simulink model "sim_tase_2025_att_ctrl"  (R2020a)
settings: Solver=ode4  StartTime=0.0  StopTime=30.0  FixedStep=0.01  RelTol=1e-3
values from neighbouring files (symbols this model uses):
  alfa_i_init = zeros(3, NF)    [init_tase_2025_att_ctrl.m]
  beta_ij_init = zeros(3, NF)    [init_tase_2025_att_ctrl.m]
  c1 = 2.5    [init_tase_2025_att_ctrl.m]
  c1_diff_sigma_bar_w = diag([12; 12; 12])    [init_tase_2025_att_ctrl.m]
  c1_diff_ui = diag([25; 30; 20])    [init_tase_2025_att_ctrl.m]
  c2 = 2.0    (= 2)    [init_tase_2025_att_ctrl.m]
  c2_diff_sigma_bar_w = diag([12; 12; 12])    [init_tase_2025_att_ctrl.m]
  c2_diff_ui = diag([50; 50; 10])    [init_tase_2025_att_ctrl.m]
  c3_diff_sigma_bar_w = diag([15; 15; 15])    [init_tase_2025_att_ctrl.m]
  c3_diff_ui = diag([15; 15; 10])    [init_tase_2025_att_ctrl.m]
  dw_aa_t = 0.2 * ones(3, 5) + ( 1.0 - 0.2 ) * rand(3, 5)    [init_tase_2025_att_ctrl.m]
  dw_ff_t = [ 0.4 * ones(1, 5) + ( 1.0 - 0.4 ) * rand(1, 5);                      0.4 * ones(1, 5) + ( 1.0 - 0.4 ) * rand(1, 5);                      0.2 * ones(1, 5) + ( 0.6 - 0.2 ) * rand(1, 5) ]    [init_tase_2025_att_ctrl.m]
  dw_phi_t = ( - pi / 2 ) * ones(3, 5) + ( pi / 2 - ( - pi / 2 ) ) * rand(3, 5)    [init_tase_2025_att_ctrl.m]
  dwci_init = zeros(3,5)    [init_tase_2025_att_ctrl.m]
  err_wi_init = zeros(3, NF)    [init_tase_2025_att_ctrl.m]
  eta_1_ij_init = zeros(3, NF)    [init_tase_2025_att_ctrl.m]
  eta_2_ij_init = zeros(3, NF)    [init_tase_2025_att_ctrl.m]
  h1w = diag([20.0; 20.0; 20.0])    [init_tase_2025_att_ctrl.m]
  h2w = diag([30.0; 35.0; 35.0])    [init_tase_2025_att_ctrl.m]
  h3w = diag([30.0; 25.0; 30.0])    [init_tase_2025_att_ctrl.m]
  Ji = zeros(3,3,NF)    [init_tase_2025_att_ctrl.m]
  k_1_ij_hat_init = zeros(3, NF)    [init_tase_2025_att_ctrl.m]
  k_1_ij_init = zeros(3, NF)    [init_tase_2025_att_ctrl.m]
  k_1_ij_lower = zeros(3, NF)    [init_tase_2025_att_ctrl.m]
  k_1_ij_upper = zeros(3, NF)    [init_tase_2025_att_ctrl.m]
  k_2_ij_init = zeros(3, NF)    [init_tase_2025_att_ctrl.m]
  k_2_ij_lower = zeros(3, NF)    [init_tase_2025_att_ctrl.m]
  k_2_ij_upper = zeros(3, NF)    [init_tase_2025_att_ctrl.m]
  Lamd_diff_sigma_bar_w = 0.8    [init_tase_2025_att_ctrl.m]
  Lamd_diff_ui = 0.8    [init_tase_2025_att_ctrl.m]
  mu1 = 0.2    [init_tase_2025_att_ctrl.m]
  mu2 = 0.2    [init_tase_2025_att_ctrl.m]
  mu_d_w = 100    [init_tase_2025_att_ctrl.m]
  phi_ij_init = ones(3, NF)    [init_tase_2025_att_ctrl.m]
  pos0 = zeros(3, 1)    [init_tase_2025_att_ctrl.m]
  PZ0 = P0(3)    [init_tase_2025_att_ctrl.m]
  PZ1 = 10    [init_tase_2025_att_ctrl.m]
  q_ij_hat_init = zeros(3, NF)    [init_tase_2025_att_ctrl.m]
  Qci_init = repmat([1;0;0;0],1,NF)    [init_tase_2025_att_ctrl.m]
  R0 = 4    [init_tase_2025_att_ctrl.m]
  R1 = 8    [init_tase_2025_att_ctrl.m]
  Rci_init = zeros(3,3,NF)    [init_tase_2025_att_ctrl.m]
  Ri_init = zeros(3,3,NF)    [init_tase_2025_att_ctrl.m]
  Rx2 = 10    [init_tase_2025_att_ctrl.m]
  Ry2 = 6    [init_tase_2025_att_ctrl.m]
  Rz2 = 4    [init_tase_2025_att_ctrl.m]
  T0 = 0    [init_tase_2025_att_ctrl.m]
  T1 = tseq1    (= 10)    [init_tase_2025_att_ctrl.m]
  T2 = tseq1 + tseq12 + tseq2    (= 30)    [init_tase_2025_att_ctrl.m]
  T_ij = repmat([60.0; 60.0; 60.0], 1, NF)    [init_tase_2025_att_ctrl.m]
  ui_init = zeros(3,NF)    [init_tase_2025_att_ctrl.m]
  vel0 = zeros(3, 1)    [init_tase_2025_att_ctrl.m]
  wci_init = zeros(3,5)    [init_tase_2025_att_ctrl.m]
  zeta_diff_sigma_bar_w = 0.3    [init_tase_2025_att_ctrl.m]
  zeta_diff_ui = 0.05    [init_tase_2025_att_ctrl.m]
undefined symbols (not defined in the file or in its folder): cal_frac_squ, p_alfaw1, p_alfaw2, q_alfaw1, q_alfaw2, Qei_init, Qi_init, Rei_init, V_Phi_Rei_init, wei_init, wi_init
(part 3 of 5)

== matlab function sim_tase_2025_att_ctrl/cal wci dwci agent 5 ==
  data: ui_vec input; wci output; duihat_vec input; d2uihat_vec input; Rci_mat input; dwci output
function [wci, dwci] = fcn(ui_vec, duihat_vec, d2uihat_vec, Rci_mat)
%%%% 计算姿态角速率指令及其导数

iiuav = 5;
ui = ui_vec(:,iiuav);
duihat = duihat_vec(:,iiuav);
d2uihat = d2uihat_vec(:,iiuav);
Rci = Rci_mat(:,:,iiuav);

ee1 = [1;0;0];
ee2 = [0;1;0];
ee3 = [0;0;1];
RciE3 = ui / norm(ui,2);
PiMat = eye(3,3) - ee3*(ee3');
dRciE3 = (1 / norm(ui,2))*Rci*PiMat*(Rci')*duihat;
Themat = [-RciE3(2)/(1+RciE3(3)),         -RciE3(1)/(1+RciE3(3)),       (RciE3(1)*RciE3(2))/((1+RciE3(3))^2); ...
                   2*RciE3(1)/(1+RciE3(3)),                0,                               1 - (RciE3(1)^2)/((1+RciE3(3))^2); ...
                               0                                       -1                                                        0                                   ];
wcxe3 = (1 / norm(ui,2))*PiMat*(Rci')*duihat;
wcxe2 = (1 / norm(ui,2))*(Rci')*Themat*Rci*PiMat*(Rci')*duihat;
wci = [-wcxe3(2); wcxe3(1); -wcxe2(1)];

TempMat1 = [0,                           -1/(1+RciE3(3)),                   (RciE3(2))/((1+RciE3(3))^2); ...
                       2/(1+RciE3(3)),                0,                               (-2*RciE3(1))/((1+RciE3(3))^2); ...
                       0,                                     0,                                                   0                             ];
TempMat2 = [-1/(1+RciE3(3)),              0,                               (RciE3(1))/((1+RciE3(3))^2); ...
                       0,                                     0,                                                   0                      ; ...
                       0,                                     0,                                                   0                             ];
TempMat3 = [(RciE3(2))/((1+RciE3(3))^2),                 (RciE3(1))/((1+RciE3(3))^2),       (-2*RciE3(1)*RciE3(2))/((1+RciE3(3))^3); ...
                       (-2*RciE3(1))/((1+RciE3(3))^2),                             0,                               (2*(RciE3(1)^2))/((1+RciE3(3))^3); ...
                        0,                                                                          0,                                                   0                             ];
dTheMat = TempMat1*dRciE3*(ee1') + TempMat2*dRciE3*(ee2') + TempMat3*dRciE3*(ee3');
wcix = cal_askew_mat(wci);
dRciT = -wcix*(Rci');
dwcxe3 = (1 / norm(ui,2))*PiMat*(dRciT*duihat+(Rci')*(d2uihat-(((ui')*duihat)/(norm(ui,2)^2))*duihat));
dwcxe2 = (1 / norm(ui,2))*((dRciT*Themat+(Rci')*dTheMat) ...
                *(Rci*PiMat*(Rci'))*duihat + (Rci')*Themat*(Rci*PiMat*(Rci'))*(d2uihat-(((ui')*duihat)/(norm(ui,2)^2))*duihat));
dwci = [-dwcxe3(2);  dwcxe3(1);  -dwcxe2(1)];

== matlab function sim_tase_2025_att_ctrl/cal alfa_i agent 1 ==
  data: c1 input; alfa_i_1 output; Qi_vec input; eta_1_ij_vec input
function alfa_i_1 = fcn(c1, Qi_vec, eta_1_ij_vec)
%%%% 计算虚拟控制量
iiuav = 1;
alfa_i_1 = -c1 * inv( (1/2) * ( Qi_vec(1,iiuav) * eye(3) + cal_askew_mat( Qi_vec(2:4,iiuav) ) ) ) * eta_1_ij_vec(:,iiuav);

== matlab function sim_tase_2025_att_ctrl/cal alfa_i agent 2 ==
  data: c1 input; alfa_i_2 output; Qi_vec input; eta_1_ij_vec input
function alfa_i_2 = fcn(c1, Qi_vec, eta_1_ij_vec)
%%%% 计算虚拟控制量
iiuav = 2;
alfa_i_2 = -c1 * inv( (1/2) * ( Qi_vec(1,iiuav) * eye(3) + cal_askew_mat( Qi_vec(2:4,iiuav) ) ) ) * eta_1_ij_vec(:,iiuav);

== matlab function sim_tase_2025_att_ctrl/cal alfa_i agent 3 ==
  data: c1 input; alfa_i_3 output; Qi_vec input; eta_1_ij_vec input
function alfa_i_3 = fcn(c1, Qi_vec, eta_1_ij_vec)
%%%% 计算虚拟控制量
iiuav = 3;
alfa_i_3 = -c1 * inv( (1/2) * ( Qi_vec(1,iiuav) * eye(3) + cal_askew_mat( Qi_vec(2:4,iiuav) ) ) ) * eta_1_ij_vec(:,iiuav);

== matlab function sim_tase_2025_att_ctrl/cal alfa_i agent 4 ==
  data: c1 input; alfa_i_4 output; Qi_vec input; eta_1_ij_vec input
function alfa_i_4 = fcn(c1, Qi_vec, eta_1_ij_vec)
%%%% 计算虚拟控制量
iiuav = 4;
alfa_i_4 = -c1 * inv( (1/2) * ( Qi_vec(1,iiuav) * eye(3) + cal_askew_mat( Qi_vec(2:4,iiuav) ) ) ) * eta_1_ij_vec(:,iiuav);

== matlab function sim_tase_2025_att_ctrl/cal alfa_i agent 5 ==
  data: c1 input; alfa_i_5 output; Qi_vec input; eta_1_ij_vec input
function alfa_i_5 = fcn(c1, Qi_vec, eta_1_ij_vec)
%%%% 计算虚拟控制量
iiuav = 5;
alfa_i_5 = -c1 * inv( (1/2) * ( Qi_vec(1,iiuav) * eye(3) + cal_askew_mat( Qi_vec(2:4,iiuav) ) ) ) * eta_1_ij_vec(:,iiuav);

== matlab function sim_tase_2025_att_ctrl/combine alfa_i ==
  data: alfa_i_1 input; alfa_i_vec output; alfa_i_2 input; alfa_i_3 input; alfa_i_4 input; alfa_i_5 input
function alfa_i_vec = fcn(alfa_i_1, alfa_i_2, alfa_i_3, alfa_i_4, alfa_i_5)
%%%% 合并预设性能函数
alfa_i_vec = [alfa_i_1(:), alfa_i_2(:), alfa_i_3(:), alfa_i_4(:), alfa_i_5(:)];

== matlab function sim_tase_2025_att_ctrl/cal phi_ij agent 1 ==
  data: tsim input; phi_ij_1 output; T_ij input
function phi_ij_1 = fcn(tsim, T_ij)
%%%% 计算性能调节函数
iiuav = 1;
phi_ij_1 = zeros(3,1);
for jj = 1:3

%     kk_phi = 1.0;
%     phi_ij_1(jj) = 1 - sin( (pi/2) * ( ( kk_phi * tsim ) / ( T_ij(jj, iiuav) ) ) );
%     if phi_ij_1(jj) < 0
%         phi_ij_1(jj) = 0;
%     end


    kk_phi = 1.0;
    if tsim <= T_ij(jj, iiuav)
        phi_ij_1(jj) = 1 - sin( (pi/2) * ( ( kk_phi * tsim ) / ( T_ij(jj, iiuav) ) ) );
    else
        phi_ij_1(jj) = 0;
    end

end

== matlab function sim_tase_2025_att_ctrl/combine wci dwci ==
  data: wci_node_1 input; wci_vec output; wci_node_2 input; wci_node_3 input; wci_node_4 input; wci_node_5 input; dwci_vec output; dwci_node_1 input; dwci_node_2 input; dwci_node_3 input; dwci_node_4 input; dwci_node_5 input
function [wci_vec, dwci_vec] = fcn(wci_node_1, wci_node_2, wci_node_3, wci_node_4, wci_node_5, ...
                                                                dwci_node_1, dwci_node_2, dwci_node_3, dwci_node_4, dwci_node_5)
%%%% 合并姿态角速率指令及其导数
wci_vec = [wci_node_1(:), wci_node_2(:), wci_node_3(:), wci_node_4(:), wci_node_5(:)];
dwci_vec = [dwci_node_1(:), dwci_node_2(:), dwci_node_3(:), dwci_node_4(:), dwci_node_5(:)];

== matlab function sim_tase_2025_att_ctrl/cal abs 11 ==
  data: x input; y output
function y = fcn(x)
y = abs(x(:));

== matlab function sim_tase_2025_att_ctrl/cal abs 12 ==
  data: x input; y output
function y = fcn(x)
y = abs(x(:));

== matlab function sim_tase_2025_att_ctrl/cal abs 13 ==
  data: x input; y output
function y = fcn(x)
y = abs(x(:));

== matlab function sim_tase_2025_att_ctrl/cal abs 14 ==
  data: x input; y output
function y = fcn(x)
y = abs(x(:));

== matlab function sim_tase_2025_att_ctrl/cal abs 15 ==
  data: x input; y output
function y = fcn(x)
y = abs(x(:));

== matlab function sim_tase_2025_att_ctrl/cal abs 16 ==
  data: x input; y output
function y = fcn(x)
y = abs(x(:));

== matlab function sim_tase_2025_att_ctrl/cal abs 17 ==
  data: x input; y output
function y = fcn(x)
y = abs(x(:));

== matlab function sim_tase_2025_att_ctrl/cal abs 18 ==
  data: x input; y output
function y = fcn(x)
y = abs(x(:));

== matlab function sim_tase_2025_att_ctrl/combine tau ==
  data: tau_1 input; taui_vec output; tau_2 input; tau_3 input; tau_4 input; tau_5 input
function taui_vec = fcn(tau_1, tau_2, tau_3, tau_4, tau_5)
%%%% 合并辅助姿态角速率
taui_vec = [tau_1(:), tau_2(:), tau_3(:), tau_4(:), tau_5(:)];

== matlab function sim_tase_2025_att_ctrl/cal phi_ij agent 2 ==
  data: tsim input; phi_ij_2 output; T_ij input
function phi_ij_2 = fcn(tsim, T_ij)
%%%% 计算性能调节函数
iiuav = 2;
phi_ij_2 = zeros(3,1);
for jj = 1:3
%     kk_phi = 1.0;
%     phi_ij_2(jj) = 1 - sin( (pi/2) * ( ( kk_phi * tsim ) / ( T_ij(jj, iiuav) ) ) );
%     if phi_ij_2(jj) < 0
%         phi_ij_2(jj) = 0;
%     end

    kk_phi = 1.0;
    if tsim <= T_ij(jj, iiuav)
        phi_ij_2(jj) = 1 - sin( (pi/2) * ( ( kk_phi * tsim ) / ( T_ij(jj, iiuav) ) ) );
    else
        phi_ij_2(jj) = 0;
    end

end

== matlab function sim_tase_2025_att_ctrl/wi dynam agent 1 ==
  data: Ji input; dwi_1 output; wi_vec input; taui_vec input; dw_vec input
function dwi_1 = fcn(Ji, wi_vec, taui_vec, dw_vec)
%%%% 更新姿态角速率微分方程
iiuav = 1;
dwi_1 = inv(Ji(:,:,iiuav)) * ( -cal_askew_mat(wi_vec(:,iiuav)) * Ji(:,:,iiuav) * wi_vec(:,iiuav) ... 
                                                + taui_vec(:,iiuav) + dw_vec(:,iiuav) );

end

== matlab function sim_tase_2025_att_ctrl/cal abs 19 ==
  data: x input; y output
function y = fcn(x)
y = abs(x(:));

== matlab function sim_tase_2025_att_ctrl/cal abs 20 ==
  data: x input; y output
function y = fcn(x)
y = abs(x(:));

== matlab function sim_tase_2025_att_ctrl/cal d_sigma_w agent 1 ==
  data: h3w input; d_sigma_w_1 output; Ji input; wi_vec input; taui_vec input; sigma_w_bar_vec input
function d_sigma_w_1 = fcn(h3w, Ji, wi_vec, taui_vec, sigma_w_bar_vec)
%%%% 计算辅助姿态角速率导数
iiuav = 1;
d_sigma_w_1 = inv(Ji(:,:,iiuav)) * ( -cal_askew_mat(wi_vec(:,iiuav)) * Ji(:,:,iiuav) * wi_vec(:,iiuav) ...
                            + taui_vec(:,iiuav) + h3w * sigma_w_bar_vec(:,iiuav) );

== matlab function sim_tase_2025_att_ctrl/cal d_sigma_w agent 2 ==
  data: h3w input; d_sigma_w_2 output; Ji input; wi_vec input; taui_vec input; sigma_w_bar_vec input
function d_sigma_w_2 = fcn(h3w, Ji, wi_vec, taui_vec, sigma_w_bar_vec)
%%%% 计算辅助姿态角速率导数
iiuav = 2;
d_sigma_w_2 = inv(Ji(:,:,iiuav)) * ( -cal_askew_mat(wi_vec(:,iiuav)) * Ji(:,:,iiuav) * wi_vec(:,iiuav) ...
                            + taui_vec(:,iiuav) + h3w * sigma_w_bar_vec(:,iiuav) );

== matlab function sim_tase_2025_att_ctrl/cal d_sigma_w agent 3 ==
  data: h3w input; d_sigma_w_3 output; Ji input; wi_vec input; taui_vec input; sigma_w_bar_vec input
function d_sigma_w_3 = fcn(h3w, Ji, wi_vec, taui_vec, sigma_w_bar_vec)
%%%% 计算辅助姿态角速率导数
iiuav = 3;
d_sigma_w_3 = inv(Ji(:,:,iiuav)) * ( -cal_askew_mat(wi_vec(:,iiuav)) * Ji(:,:,iiuav) * wi_vec(:,iiuav) ...
                            + taui_vec(:,iiuav) + h3w * sigma_w_bar_vec(:,iiuav) );

== matlab function sim_tase_2025_att_ctrl/cal d_sigma_w agent 4 ==
  data: h3w input; d_sigma_w_4 output; Ji input; wi_vec input; taui_vec input; sigma_w_bar_vec input
function d_sigma_w_4 = fcn(h3w, Ji, wi_vec, taui_vec, sigma_w_bar_vec)
%%%% 计算辅助姿态角速率导数
iiuav = 4;
d_sigma_w_4 = inv(Ji(:,:,iiuav)) * ( -cal_askew_mat(wi_vec(:,iiuav)) * Ji(:,:,iiuav) * wi_vec(:,iiuav) ...
                            + taui_vec(:,iiuav) + h3w * sigma_w_bar_vec(:,iiuav) );

== matlab function sim_tase_2025_att_ctrl/wi dynam agent 2 ==
  data: Ji input; dwi_2 output; wi_vec input; taui_vec input; dw_vec input
function dwi_2 = fcn(Ji, wi_vec, taui_vec, dw_vec)
%%%% 更新姿态角速率微分方程
iiuav = 2;
dwi_2 = inv(Ji(:,:,iiuav)) * ( -cal_askew_mat(wi_vec(:,iiuav)) * Ji(:,:,iiuav) * wi_vec(:,iiuav) ... 
                                                + taui_vec(:,iiuav) + dw_vec(:,iiuav) );

end

== matlab function sim_tase_2025_att_ctrl/cal phi_ij agent 3 ==
  data: tsim input; phi_ij_3 output; T_ij input
function phi_ij_3 = fcn(tsim, T_ij)
%%%% 计算性能调节函数
iiuav = 3;
phi_ij_3 = zeros(3,1);
for jj = 1:3
%     kk_phi = 1.0;
%     phi_ij_3(jj) = 1 - sin( (pi/2) * ( ( kk_phi * tsim ) / ( T_ij(jj, iiuav) ) ) );
%     if phi_ij_3(jj) < 0
%         phi_ij_3(jj) = 0;
%     end

    kk_phi = 1.0;
    if tsim <= T_ij(jj, iiuav)
        phi_ij_3(jj) = 1 - sin( (pi/2) * ( ( kk_phi * tsim ) / ( T_ij(jj, iiuav) ) ) );
    else
        phi_ij_3(jj) = 0;
    end

end

== matlab function sim_tase_2025_att_ctrl/wi dynam agent 3 ==
  data: Ji input; dwi_3 output; wi_vec input; taui_vec input; dw_vec input
function dwi_3 = fcn(Ji, wi_vec, taui_vec, dw_vec)
%%%% 更新姿态角速率微分方程
iiuav = 3;
dwi_3 = inv(Ji(:,:,iiuav)) * ( -cal_askew_mat(wi_vec(:,iiuav)) * Ji(:,:,iiuav) * wi_vec(:,iiuav) ...
                                                + taui_vec(:,iiuav) + dw_vec(:,iiuav) );

end

== matlab function sim_tase_2025_att_ctrl/wi dynam agent 4 ==
  data: Ji input; dwi_4 output; wi_vec input; taui_vec input; dw_vec input
function dwi_4 = fcn(Ji, wi_vec, taui_vec, dw_vec)
%%%% 更新姿态角速率微分方程
iiuav = 4;
dwi_4 = inv(Ji(:,:,iiuav)) * ( -cal_askew_mat(wi_vec(:,iiuav)) * Ji(:,:,iiuav) * wi_vec(:,iiuav) ...
                                                + taui_vec(:,iiuav) + dw_vec(:,iiuav) );

end

== matlab function sim_tase_2025_att_ctrl/wi dynam agent 5 ==
  data: Ji input; dwi_5 output; wi_vec input; taui_vec input; dw_vec input
function dwi_5 = fcn(Ji, wi_vec, taui_vec, dw_vec)
%%%% 更新姿态角速率微分方程
iiuav = 5;
dwi_5 = inv(Ji(:,:,iiuav)) * ( -cal_askew_mat(wi_vec(:,iiuav)) * Ji(:,:,iiuav) * wi_vec(:,iiuav) ...
                                                + taui_vec(:,iiuav) + dw_vec(:,iiuav) );

end

== matlab function sim_tase_2025_att_ctrl/combine dwi ==
  data: wi_1 input; wi_vec output; wi_2 input; wi_3 input; wi_4 input; wi_5 input
function wi_vec = fcn(wi_1, wi_2, wi_3, wi_4, wi_5)
%%%% 合并姿态角速率
wi_vec = [wi_1(:), wi_2(:), wi_3(:), wi_4(:), wi_5(:)];

== matlab function sim_tase_2025_att_ctrl/Qi dynam agent 1 ==
  data: Qi_vec input; dQi_1 output; wi_vec input
function dQi_1 = fcn(Qi_vec, wi_vec)
%%%% 更新四元数微分方程
iiuav = 1;

wi = wi_vec(:,iiuav);
thetai = Qi_vec(1,iiuav);
qi = Qi_vec(2:4,iiuav);

GammaQi = zeros(4,3);
GammaQi(1,:) = -(qi');
GammaQi(2:4,:) = thetai*eye(3,3) + cal_askew_mat(qi);
dQi_1 = (1/2)*GammaQi*wi;

end

== matlab function sim_tase_2025_att_ctrl/Qi dynam agent 2 ==
  data: Qi_vec input; dQi_2 output; wi_vec input
function dQi_2 = fcn(Qi_vec, wi_vec)
%%%% 更新四元数微分方程
iiuav = 2;

wi = wi_vec(:,iiuav);
thetai = Qi_vec(1,iiuav);
qi = Qi_vec(2:4,iiuav);

GammaQi = zeros(4,3);
GammaQi(1,:) = -(qi');
GammaQi(2:4,:) = thetai*eye(3,3) + cal_askew_mat(qi);
dQi_2 = (1/2)*GammaQi*wi;

end

== matlab function sim_tase_2025_att_ctrl/cal d_sigma_w agent 5 ==
  data: h3w input; d_sigma_w_5 output; Ji input; wi_vec input; taui_vec input; sigma_w_bar_vec input
function d_sigma_w_5 = fcn(h3w, Ji, wi_vec, taui_vec, sigma_w_bar_vec)
%%%% 计算辅助姿态角速率导数
iiuav = 5;
d_sigma_w_5 = inv(Ji(:,:,iiuav)) * ( -cal_askew_mat(wi_vec(:,iiuav)) * Ji(:,:,iiuav) * wi_vec(:,iiuav) ...
                            + taui_vec(:,iiuav) + h3w * sigma_w_bar_vec(:,iiuav) );

== matlab function sim_tase_2025_att_ctrl/cal differentiator d_sigma_bar_w_hat agent 1/cal differentiator ==
  data: c1 input; d_sigma_bar_v_hat output; d_dsigma_bar_v_hat output; d_d2sigma_bar_v_hat output; c2 input; c3 input; chi_t input; sigma_bar_v_sig_1 input; sigma_bar_v_sig_2 input; sigma_bar_v_sig_3 input; sigma_bar_v_sig_4 input; sigma_bar_v_sig_5 input; sigma_bar_v_sig_6 input; d_sigma_bar_v_hat input; d2_sigma_bar_v_hat input
function [d_sigma_bar_v_hat, d_dsigma_bar_v_hat, d_d2sigma_bar_v_hat] = fcn(c1, c2, c3, chi_t, sigma_bar_v_sig_1, sigma_bar_v_sig_2, sigma_bar_v_sig_3, ...
                                                                                                                                                sigma_bar_v_sig_4, sigma_bar_v_sig_5, sigma_bar_v_sig_6, d_sigma_bar_v_hat, d2_sigma_bar_v_hat)
d_d2sigma_bar_v_hat = -chi_t .* c1 * sigma_bar_v_sig_1(:) - (1 - chi_t) .* c1 * sigma_bar_v_sig_2(:);
d_dsigma_bar_v_hat = -chi_t .* c2 * sigma_bar_v_sig_3(:) - (1 - chi_t) .* c2 * sigma_bar_v_sig_4(:) + d2_sigma_bar_v_hat(:);
d_sigma_bar_v_hat = -chi_t .* c3 * sigma_bar_v_sig_5(:) - (1 - chi_t) .* c3 * sigma_bar_v_sig_6(:) + d_sigma_bar_v_hat(:);

== matlab function sim_tase_2025_att_ctrl/cal phi_ij agent 4 ==
  data: tsim input; phi_ij_4 output; T_ij input
function phi_ij_4 = fcn(tsim, T_ij)
%%%% 计算性能调节函数
iiuav = 4;
phi_ij_4 = zeros(3,1);
for jj = 1:3
%     kk_phi = 1.0;
%     phi_ij_4(jj) = 1 - sin( (pi/2) * ( ( kk_phi * tsim ) / ( T_ij(jj, iiuav) ) ) );
%     if phi_ij_4(jj) < 0
%         phi_ij_4(jj) = 0;
%     end

    kk_phi = 1.0;
    if tsim <= T_ij(jj, iiuav)
        phi_ij_4(jj) = 1 - sin( (pi/2) * ( ( kk_phi * tsim ) / ( T_ij(jj, iiuav) ) ) );
    else
        phi_ij_4(jj) = 0;
    end

end

== matlab function sim_tase_2025_att_ctrl/cal differentiator d_sigma_bar_w_hat agent 1/cal sig ==
  data: x input; z output; y input
function z = fcn(x, y)
z = x(:) .* sign(y(:));

== matlab function sim_tase_2025_att_ctrl/cal differentiator d_sigma_bar_w_hat agent 1/cal sig1 ==
  data: x input; z output; y input
function z = fcn(x, y)
z = x(:) .* sign(y(:));

== matlab function sim_tase_2025_att_ctrl/cal differentiator d_sigma_bar_w_hat agent 1/cal sig2 ==
  data: x input; z output; y input
function z = fcn(x, y)
z = x(:) .* sign(y(:));

== matlab function sim_tase_2025_att_ctrl/cal differentiator d_sigma_bar_w_hat agent 1/cal sig3 ==
  data: x input; z output; y input
function z = fcn(x, y)
z = x(:) .* sign(y(:));

== matlab function sim_tase_2025_att_ctrl/cal differentiator d_sigma_bar_w_hat agent 1/cal sig4 ==
  data: x input; z output; y input
function z = fcn(x, y)
z = x(:) .* sign(y(:));

== matlab function sim_tase_2025_att_ctrl/cal differentiator d_sigma_bar_w_hat agent 1/cal sig5 ==
  data: x input; z output; y input
function z = fcn(x, y)
z = x(:) .* sign(y(:));

== matlab function sim_tase_2025_att_ctrl/cal differentiator d_sigma_bar_w_hat agent 1/choose sigma_bar_w ==
  data: x input; y output
function y = fcn(x)
iiuav = 1;
y = x(:,iiuav);

== matlab function sim_tase_2025_att_ctrl/cal differentiator d_sigma_bar_w_hat agent 1/trans to column20 ==
  data: x input; y output
function y = fcn(x)
y = x(:);

== matlab function sim_tase_2025_att_ctrl/cal differentiator d_sigma_bar_w_hat agent 1/trans to column21 ==
  data: x input; y output
function y = fcn(x)
y = x(:);

== matlab function sim_tase_2025_att_ctrl/depart wc5 ==
  data: y output; x input
function y = fcn(x)
y = x(:,5);

end

== matlab function sim_tase_2025_att_ctrl/cal differentiator d_sigma_bar_w_hat agent 1/trans to column22 ==
  data: x input; y output
function y = fcn(x)
y = x(:);

== matlab function sim_tase_2025_att_ctrl/cal differentiator d_sigma_bar_w_hat agent 1/trans to column23 ==
  data: x input; y output
function y = fcn(x)
y = x(:);

== matlab function sim_tase_2025_att_ctrl/cal differentiator d_sigma_bar_w_hat agent 1/trans to column24 ==
  data: x input; y output
function y = fcn(x)
y = x(:);

== matlab function sim_tase_2025_att_ctrl/cal differentiator d_sigma_bar_w_hat agent 1/trans to column25 ==
  data: x input; y output
function y = fcn(x)
y = x(:);

== matlab function sim_tase_2025_att_ctrl/cal differentiator d_sigma_bar_w_hat agent 2/cal differentiator ==
  data: c1 input; d_sigma_bar_v_hat output; d_dsigma_bar_v_hat output; d_d2sigma_bar_v_hat output; c2 input; c3 input; chi_t input; sigma_bar_v_sig_1 input; sigma_bar_v_sig_2 input; sigma_bar_v_sig_3 input; sigma_bar_v_sig_4 input; sigma_bar_v_sig_5 input; sigma_bar_v_sig_6 input; d_sigma_bar_v_hat input; d2_sigma_bar_v_hat input
function [d_sigma_bar_v_hat, d_dsigma_bar_v_hat, d_d2sigma_bar_v_hat] = fcn(c1, c2, c3, chi_t, sigma_bar_v_sig_1, sigma_bar_v_sig_2, sigma_bar_v_sig_3, ...
                                                                                                                                                sigma_bar_v_sig_4, sigma_bar_v_sig_5, sigma_bar_v_sig_6, d_sigma_bar_v_hat, d2_sigma_bar_v_hat)
d_d2sigma_bar_v_hat = -chi_t .* c1 * sigma_bar_v_sig_1(:) - (1 - chi_t) .* c1 * sigma_bar_v_sig_2(:);
d_dsigma_bar_v_hat = -chi_t .* c2 * sigma_bar_v_sig_3(:) - (1 - chi_t) .* c2 * sigma_bar_v_sig_4(:) + d2_sigma_bar_v_hat(:);
d_sigma_bar_v_hat = -chi_t .* c3 * sigma_bar_v_sig_5(:) - (1 - chi_t) .* c3 * sigma_bar_v_sig_6(:) + d_sigma_bar_v_hat(:);

== matlab function sim_tase_2025_att_ctrl/cal differentiator d_sigma_bar_w_hat agent 2/cal sig ==
  data: x input; z output; y input
function z = fcn(x, y)
z = x(:) .* sign(y(:));

== matlab function sim_tase_2025_att_ctrl/cal differentiator d_sigma_bar_w_hat agent 2/cal sig1 ==
  data: x input; z output; y input
function z = fcn(x, y)
z = x(:) .* sign(y(:));

== matlab function sim_tase_2025_att_ctrl/cal differentiator d_sigma_bar_w_hat agent 2/cal sig2 ==
  data: x input; z output; y input
function z = fcn(x, y)
z = x(:) .* sign(y(:));

== matlab function sim_tase_2025_att_ctrl/depart wc1 ==
  data: y output; x input
function y = fcn(x)
y = x(:,1);

end

== matlab function sim_tase_2025_att_ctrl/cal differentiator d_sigma_bar_w_hat agent 2/cal sig3 ==
  data: x input; z output; y input
function z = fcn(x, y)
z = x(:) .* sign(y(:));

== matlab function sim_tase_2025_att_ctrl/cal differentiator d_sigma_bar_w_hat agent 2/cal sig4 ==
  data: x input; z output; y input
function z = fcn(x, y)
z = x(:) .* sign(y(:));

== matlab function sim_tase_2025_att_ctrl/cal differentiator d_sigma_bar_w_hat agent 2/cal sig5 ==
  data: x input; z output; y input
function z = fcn(x, y)
z = x(:) .* sign(y(:));

== matlab function sim_tase_2025_att_ctrl/cal differentiator d_sigma_bar_w_hat agent 2/choose sigma_bar_w ==
  data: x input; y output
function y = fcn(x)
iiuav = 2;
y = x(:,iiuav);

== matlab function sim_tase_2025_att_ctrl/cal differentiator d_sigma_bar_w_hat agent 2/trans to column20 ==
  data: x input; y output
function y = fcn(x)
y = x(:);

== matlab function sim_tase_2025_att_ctrl/cal differentiator d_sigma_bar_w_hat agent 2/trans to column21 ==
  data: x input; y output
function y = fcn(x)
y = x(:);

== matlab function sim_tase_2025_att_ctrl/cal differentiator d_sigma_bar_w_hat agent 2/trans to column22 ==
  data: x input; y output
function y = fcn(x)
y = x(:);

== matlab function sim_tase_2025_att_ctrl/cal differentiator d_sigma_bar_w_hat agent 2/trans to column23 ==
  data: x input; y output
function y = fcn(x)
y = x(:);

== matlab function sim_tase_2025_att_ctrl/cal taui agent 1 ==
  data: c2 input; beta_i_vec input; eta_2_ij_vec input; tau_1 output; dw_hat_vec input
function tau_1 = fcn(c2, beta_i_vec, eta_2_ij_vec, dw_hat_vec)
%%%% 计算用于姿态控制的驱动力矩控制输入
iiuav = 1;
tau_1 = -c2 * beta_i_vec(:,iiuav) .* eta_2_ij_vec(:,iiuav) - dw_hat_vec(:,iiuav);
end

== matlab function sim_tase_2025_att_ctrl/depart wc2 ==
  data: y output; x input
function y = fcn(x)
y = x(:,2);

end

== matlab function sim_tase_2025_att_ctrl/Qi dynam agent 3 ==
  data: Qi_vec input; dQi_3 output; wi_vec input
function dQi_3 = fcn(Qi_vec, wi_vec)
%%%% 更新四元数微分方程
iiuav = 3;

wi = wi_vec(:,iiuav);
thetai = Qi_vec(1,iiuav);
qi = Qi_vec(2:4,iiuav);

GammaQi = zeros(4,3);
GammaQi(1,:) = -(qi');
GammaQi(2:4,:) = thetai*eye(3,3) + cal_askew_mat(qi);
dQi_3 = (1/2)*GammaQi*wi;

end

== matlab function sim_tase_2025_att_ctrl/Qi dynam agent 4 ==
  data: Qi_vec input; dQi_4 output; wi_vec input
function dQi_4 = fcn(Qi_vec, wi_vec)
%%%% 更新四元数微分方程
iiuav = 4;

wi = wi_vec(:,iiuav);
thetai = Qi_vec(1,iiuav);
qi = Qi_vec(2:4,iiuav);

GammaQi = zeros(4,3);
GammaQi(1,:) = -(qi');
GammaQi(2:4,:) = thetai*eye(3,3) + cal_askew_mat(qi);
dQi_4 = (1/2)*GammaQi*wi;

end

== matlab function sim_tase_2025_att_ctrl/Qi dynam agent 5 ==
  data: Qi_vec input; dQi_5 output; wi_vec input
function dQi_5 = fcn(Qi_vec, wi_vec)
%%%% 更新四元数微分方程
iiuav = 5;

wi = wi_vec(:,iiuav);
thetai = Qi_vec(1,iiuav);
qi = Qi_vec(2:4,iiuav);

GammaQi = zeros(4,3);
GammaQi(1,:) = -(qi');
GammaQi(2:4,:) = thetai*eye(3,3) + cal_askew_mat(qi);
dQi_5 = (1/2)*GammaQi*wi;

end

== matlab function sim_tase_2025_att_ctrl/combine Qi Ri ==
  data: Qi_1 input; Qi_vec output; Qi_2 input; Qi_3 input; Qi_4 input; Qi_5 input; Ri_1 input; Ri_2 input; Ri_3 input; Ri_4 input; Ri_5 input; Ri_vec output
function [Qi_vec, Ri_vec] = fcn(Qi_1, Qi_2, Qi_3, Qi_4, Qi_5, ...
                                                        Ri_1, Ri_2, Ri_3, Ri_4, Ri_5)
%%%% 合并四元数和姿态旋转矩阵
Qi_vec = zeros(4,5);
Qi_vec(:,1) = Qi_1(:);
Qi_vec(:,2) = Qi_2(:);
Qi_vec(:,3) = Qi_3(:);
Qi_vec(:,4) = Qi_4(:);
Qi_vec(:,5) = Qi_5(:);

Ri_vec = zeros(3,3,5);
Ri_vec(:,:,1) = Ri_1;
Ri_vec(:,:,2) = Ri_2;
Ri_vec(:,:,3) = Ri_3;
Ri_vec(:,:,4) = Ri_4;
Ri_vec(:,:,5) = Ri_5;

== matlab function sim_tase_2025_att_ctrl/cal differentiator d_sigma_bar_w_hat agent 2/trans to column24 ==
  data: x input; y output
function y = fcn(x)
y = x(:);

== matlab function sim_tase_2025_att_ctrl/cal differentiator d_sigma_bar_w_hat agent 2/trans to column25 ==
  data: x input; y output
function y = fcn(x)
y = x(:);

== matlab function sim_tase_2025_att_ctrl/cal differentiator d_sigma_bar_w_hat agent 3/cal differentiator ==
  data: c1 input; d_sigma_bar_v_hat output; d_dsigma_bar_v_hat output; d_d2sigma_bar_v_hat output; c2 input; c3 input; chi_t input; sigma_bar_v_sig_1 input; sigma_bar_v_sig_2 input; sigma_bar_v_sig_3 input; sigma_bar_v_sig_4 input; sigma_bar_v_sig_5 input; sigma_bar_v_sig_6 input; d_sigma_bar_v_hat input; d2_sigma_bar_v_hat input
function [d_sigma_bar_v_hat, d_dsigma_bar_v_hat, d_d2sigma_bar_v_hat] = fcn(c1, c2, c3, chi_t, sigma_bar_v_sig_1, sigma_bar_v_sig_2, sigma_bar_v_sig_3, ...
                                                                                                                                                sigma_bar_v_sig_4, sigma_bar_v_sig_5, sigma_bar_v_sig_6, d_sigma_bar_v_hat, d2_sigma_bar_v_hat)
d_d2sigma_bar_v_hat = -chi_t .* c1 * sigma_bar_v_sig_1(:) - (1 - chi_t) .* c1 * sigma_bar_v_sig_2(:);
d_dsigma_bar_v_hat = -chi_t .* c2 * sigma_bar_v_sig_3(:) - (1 - chi_t) .* c2 * sigma_bar_v_sig_4(:) + d2_sigma_bar_v_hat(:);
d_sigma_bar_v_hat = -chi_t .* c3 * sigma_bar_v_sig_5(:) - (1 - chi_t) .* c3 * sigma_bar_v_sig_6(:) + d_sigma_bar_v_hat(:);

== matlab function sim_tase_2025_att_ctrl/depart wc3 ==
  data: y output; x input
function y = fcn(x)
y = x(:,3);

end

== matlab function sim_tase_2025_att_ctrl/cal differentiator d_sigma_bar_w_hat agent 3/cal sig ==
  data: x input; z output; y input
function z = fcn(x, y)
z = x(:) .* sign(y(:));

== matlab function sim_tase_2025_att_ctrl/cal differentiator d_sigma_bar_w_hat agent 3/cal sig1 ==
  data: x input; z output; y input
function z = fcn(x, y)
z = x(:) .* sign(y(:));

== matlab function sim_tase_2025_att_ctrl/cal err_wi agent 1 ==
  data: wi_vec input; err_wi_1 output; alfa_i_vec input
function err_wi_1 = fcn(wi_vec, alfa_i_vec)
%%%% 计算姿态角速率虚拟跟踪误差
iiuav = 1;
err_wi_1 = wi_vec(:,iiuav) - alfa_i_vec(:,iiuav);

== matlab function sim_tase_2025_att_ctrl/cal differentiator d_sigma_bar_w_hat agent 3/cal sig2 ==
  data: x input; z output; y input
function z = fcn(x, y)
z = x(:) .* sign(y(:));

== matlab function sim_tase_2025_att_ctrl/cal err_wi agent 2 ==
  data: wi_vec input; err_wi_2 output; alfa_i_vec input
function err_wi_2 = fcn(wi_vec, alfa_i_vec)
%%%% 计算姿态角速率虚拟跟踪误差
iiuav = 2;
err_wi_2 = wi_vec(:,iiuav) - alfa_i_vec(:,iiuav);

== matlab function sim_tase_2025_att_ctrl/cal err_wi agent 3 ==
  data: wi_vec input; err_wi_3 output; alfa_i_vec input
function err_wi_3 = fcn(wi_vec, alfa_i_vec)
%%%% 计算姿态角速率虚拟跟踪误差
iiuav = 3;
err_wi_3 = wi_vec(:,iiuav) - alfa_i_vec(:,iiuav);

== matlab function sim_tase_2025_att_ctrl/cal err_wi agent 4 ==
  data: wi_vec input; err_wi_4 output; alfa_i_vec input
function err_wi_4 = fcn(wi_vec, alfa_i_vec)
%%%% 计算姿态角速率虚拟跟踪误差
iiuav = 4;
err_wi_4 = wi_vec(:,iiuav) - alfa_i_vec(:,iiuav);

== matlab function sim_tase_2025_att_ctrl/cal err_wi agent 5 ==
  data: wi_vec input; err_wi_5 output; alfa_i_vec input
function err_wi_5 = fcn(wi_vec, alfa_i_vec)
%%%% 计算姿态角速率虚拟跟踪误差
iiuav = 5;
err_wi_5 = wi_vec(:,iiuav) - alfa_i_vec(:,iiuav);

== matlab function sim_tase_2025_att_ctrl/depart wc4 ==
  data: y output; x input
function y = fcn(x)
y = x(:,4);

end

== matlab function sim_tase_2025_att_ctrl/combine err_wi ==
  data: err_wi_1 input; err_wi_vec output; err_wi_2 input; err_wi_3 input; err_wi_4 input; err_wi_5 input
function err_wi_vec = fcn(err_wi_1, err_wi_2, err_wi_3, err_wi_4, err_wi_5)
%%%% 合并姿态角速率虚拟跟踪误差
err_wi_vec = [err_wi_1(:), err_wi_2(:), err_wi_3(:), err_wi_4(:), err_wi_5(:)];

== matlab function sim_tase_2025_att_ctrl/cal k_2_ij agent 1 ==
  data: mu2 input; k_2_ij_upper input; k_2_ij_lower input; k_2_ij_node_1 output; tsim input
function k_2_ij_node_1 = fcn(mu2, k_2_ij_upper, k_2_ij_lower, tsim)
%%%% 计算预设性能函数
iiuav = 1;
k_2_ij_node_1 = zeros(3,1);
for jj = 1:3
    k_2_ij_node_1(jj) = k_2_ij_lower(jj,iiuav) + ( k_2_ij_upper(jj,iiuav) - k_2_ij_lower(jj,iiuav) ) * exp( -mu2 * tsim );
end

== matlab function sim_tase_2025_att_ctrl/cal k_2_ij agent 2 ==
  data: mu2 input; k_2_ij_upper input; k_2_ij_lower input; k_2_ij_node_2 output; tsim input
function k_2_ij_node_2 = fcn(mu2, k_2_ij_upper, k_2_ij_lower, tsim)
%%%% 计算预设性能函数
iiuav = 2;
k_2_ij_node_2 = zeros(3,1);
for jj = 1:3
    k_2_ij_node_2(jj) = k_2_ij_lower(jj,iiuav) + ( k_2_ij_upper(jj,iiuav) - k_2_ij_lower(jj,iiuav) ) * exp( -mu2 * tsim );
end

== matlab function sim_tase_2025_att_ctrl/depart k_1_ij 5 ==
  data: y output; x input
function y = fcn(x)
y = x(:,5);

end

== matlab function sim_tase_2025_att_ctrl/cal k_2_ij agent 3 ==
  data: mu2 input; k_2_ij_upper input; k_2_ij_lower input; k_2_ij_node_3 output; tsim input
function k_2_ij_node_3 = fcn(mu2, k_2_ij_upper, k_2_ij_lower, tsim)
%%%% 计算预设性能函数
iiuav = 3;
k_2_ij_node_3 = zeros(3,1);
for jj = 1:3
    k_2_ij_node_3(jj) = k_2_ij_lower(jj,iiuav) + ( k_2_ij_upper(jj,iiuav) - k_2_ij_lower(jj,iiuav) ) * exp( -mu2 * tsim );
end

== matlab function sim_tase_2025_att_ctrl/depart k_1_ij 1 ==
  data: y output; x input
function y = fcn(x)
y = x(:,1);

end

== matlab function sim_tase_2025_att_ctrl/depart k_1_ij 2 ==
  data: y output; x input
function y = fcn(x)
y = x(:,2);

end

== matlab function sim_tase_2025_att_ctrl/depart k_1_ij 3 ==
  data: y output; x input
function y = fcn(x)
y = x(:,3);

end

== matlab function sim_tase_2025_att_ctrl/depart Qc5 ==
  data: y output; x input
function y = fcn(x)
y = x(:,5);

end

== matlab function sim_tase_2025_att_ctrl/cal k_2_ij agent 4 ==
  data: mu2 input; k_2_ij_upper input; k_2_ij_lower input; k_2_ij_node_4 output; tsim input
function k_2_ij_node_4 = fcn(mu2, k_2_ij_upper, k_2_ij_lower, tsim)
%%%% 计算预设性能函数
iiuav = 4;
k_2_ij_node_4 = zeros(3,1);
for jj = 1:3
    k_2_ij_node_4(jj) = k_2_ij_lower(jj,iiuav) + ( k_2_ij_upper(jj,iiuav) - k_2_ij_lower(jj,iiuav) ) * exp( -mu2 * tsim );
end

== matlab function sim_tase_2025_att_ctrl/cal k_2_ij agent 5 ==
  data: mu2 input; k_2_ij_upper input; k_2_ij_lower input; k_2_ij_node_5 output; tsim input
function k_2_ij_node_5 = fcn(mu2, k_2_ij_upper, k_2_ij_lower, tsim)
%%%% 计算预设性能函数
iiuav = 5;
k_2_ij_node_5 = zeros(3,1);
for jj = 1:3
    k_2_ij_node_5(jj) = k_2_ij_lower(jj,iiuav) + ( k_2_ij_upper(jj,iiuav) - k_2_ij_lower(jj,iiuav) ) * exp( -mu2 * tsim );
end

== matlab function sim_tase_2025_att_ctrl/combine k_2_ij ==
  data: k_2_ij_node_1 input; k_2_ij_vec output; k_2_ij_node_2 input; k_2_ij_node_3 input; k_2_ij_node_4 input; k_2_ij_node_5 input
function k_2_ij_vec = fcn(k_2_ij_node_1, k_2_ij_node_2, k_2_ij_node_3, k_2_ij_node_4, k_2_ij_node_5)
%%%% 合并预设性能函数
k_2_ij_vec = [k_2_ij_node_1(:), k_2_ij_node_2(:), k_2_ij_node_3(:), k_2_ij_node_4(:), k_2_ij_node_5(:)];

== matlab function sim_tase_2025_att_ctrl/cal eta_2_ij agent 1 ==
  data: k_2_ij_vec input; err_wi_vec input; eta_2_ij_node_1 output
function eta_2_ij_node_1 = fcn(k_2_ij_vec, err_wi_vec)
%%%% 计算障碍函数
iiuav = 1;
eta_2_ij_node_1 = zeros(3,1);
for jj = 1:3
    eta_2_ij_node_1(jj) = tan( (pi/2) * ( err_wi_vec(jj,iiuav) / k_2_ij_vec(jj,iiuav) ) );
end

== matlab function sim_tase_2025_att_ctrl/cal eta_2_ij agent 2 ==
  data: k_2_ij_vec input; err_wi_vec input; eta_2_ij_node_2 output
function eta_2_ij_node_2 = fcn(k_2_ij_vec, err_wi_vec)
%%%% 计算障碍函数
iiuav = 2;
eta_2_ij_node_2 = zeros(3,1);
for jj = 1:3
    eta_2_ij_node_2(jj) = tan( (pi/2) * ( err_wi_vec(jj,iiuav) / k_2_ij_vec(jj,iiuav) ) );
end

== matlab function sim_tase_2025_att_ctrl/cal eta_2_ij agent 3 ==
  data: k_2_ij_vec input; err_wi_vec input; eta_2_ij_node_3 output
function eta_2_ij_node_3 = fcn(k_2_ij_vec, err_wi_vec)
%%%% 计算障碍函数
iiuav = 3;
eta_2_ij_node_3 = zeros(3,1);
for jj = 1:3
    eta_2_ij_node_3(jj) = tan( (pi/2) * ( err_wi_vec(jj,iiuav) / k_2_ij_vec(jj,iiuav) ) );
end

== matlab function sim_tase_2025_att_ctrl/cal eta_2_ij agent 4 ==
  data: k_2_ij_vec input; err_wi_vec input; eta_2_ij_node_4 output
function eta_2_ij_node_4 = fcn(k_2_ij_vec, err_wi_vec)
%%%% 计算障碍函数
iiuav = 4;
eta_2_ij_node_4 = zeros(3,1);
for jj = 1:3
    eta_2_ij_node_4(jj) = tan( (pi/2) * ( err_wi_vec(jj,iiuav) / k_2_ij_vec(jj,iiuav) ) );
end

== matlab function sim_tase_2025_att_ctrl/cal eta_2_ij agent 5 ==
  data: k_2_ij_vec input; err_wi_vec input; eta_2_ij_node_5 output
function eta_2_ij_node_5 = fcn(k_2_ij_vec, err_wi_vec)
%%%% 计算障碍函数
iiuav = 5;
eta_2_ij_node_5 = zeros(3,1);
for jj = 1:3
    eta_2_ij_node_5(jj) = tan( (pi/2) * ( err_wi_vec(jj,iiuav) / k_2_ij_vec(jj,iiuav) ) );
end

== matlab function sim_tase_2025_att_ctrl/depart Qc1 ==
  data: y output; x input
function y = fcn(x)
y = x(:,1);

end

== matlab function sim_tase_2025_att_ctrl/combine eta_2_ij ==
  data: eta_2_ij_node_1 input; eta_2_ij_vec output; eta_2_ij_node_2 input; eta_2_ij_node_3 input; eta_2_ij_node_4 input; eta_2_ij_node_5 input
function eta_2_ij_vec = fcn(eta_2_ij_node_1, eta_2_ij_node_2, eta_2_ij_node_3, eta_2_ij_node_4, eta_2_ij_node_5)
%%%% 合并预设性能函数
eta_2_ij_vec = [eta_2_ij_node_1(:), eta_2_ij_node_2(:), eta_2_ij_node_3(:), eta_2_ij_node_4(:), eta_2_ij_node_5(:)];

== matlab function sim_tase_2025_att_ctrl/cal beta_i agent 1 ==
  data: k_2_ij_vec input; err_wi_vec input; beta_i_node_1 output
function beta_i_node_1 = fcn(k_2_ij_vec, err_wi_vec)
%%%% 计算障碍函数偏导数
iiuav = 1;
beta_i_node_1 = zeros(3,1);
for jj = 1:3
%     beta_i_node_1(jj) = ( 1 / k_2_ij_vec(jj,iiuav) ) * ( 1 / ( cos( (pi/2) * ( err_wi_vec(jj,iiuav) / k_2_ij_vec(jj,iiuav) ) ) ^ 2 ) );
    beta_i_node_1(jj) = ( 1 / k_2_ij_vec(jj,iiuav) ) * ( pi / 2 ) * ( 1 / ( cos( (pi/2) * ( err_wi_vec(jj,iiuav) / k_2_ij_vec(jj,iiuav) ) ) ^ 2 ) );
end

== matlab function sim_tase_2025_att_ctrl/cal beta_i agent 2 ==
  data: k_2_ij_vec input; err_wi_vec input; beta_i_node_2 output
function beta_i_node_2 = fcn(k_2_ij_vec, err_wi_vec)
%%%% 计算障碍函数偏导数
iiuav = 2;
beta_i_node_2 = zeros(3,1);
for jj = 1:3
%     beta_i_node_2(jj) = ( 1 / k_2_ij_vec(jj,iiuav) ) * ( 1 / ( cos( (pi/2) * ( err_wi_vec(jj,iiuav) / k_2_ij_vec(jj,iiuav) ) ) ^ 2 ) );
    beta_i_node_2(jj) = ( 1 / k_2_ij_vec(jj,iiuav) ) * ( pi / 2 ) * ( 1 / ( cos( (pi/2) * ( err_wi_vec(jj,iiuav) / k_2_ij_vec(jj,iiuav) ) ) ^ 2 ) );
end

== matlab function sim_tase_2025_att_ctrl/cal beta_i agent 3 ==
  data: k_2_ij_vec input; err_wi_vec input; beta_i_node_3 output
function beta_i_node_3 = fcn(k_2_ij_vec, err_wi_vec)
%%%% 计算障碍函数偏导数
iiuav = 3;
beta_i_node_3 = zeros(3,1);
for jj = 1:3
%     beta_i_node_3(jj) = ( 1 / k_2_ij_vec(jj,iiuav) ) * ( 1 / ( cos( (pi/2) * ( err_wi_vec(jj,iiuav) / k_2_ij_vec(jj,iiuav) ) ) ^ 2 ) );
    beta_i_node_3(jj) = ( 1 / k_2_ij_vec(jj,iiuav) ) * ( pi / 2 ) * ( 1 / ( cos( (pi/2) * ( err_wi_vec(jj,iiuav) / k_2_ij_vec(jj,iiuav) ) ) ^ 2 ) );
end

== matlab function sim_tase_2025_att_ctrl/cal beta_i agent 4 ==
  data: k_2_ij_vec input; err_wi_vec input; beta_i_node_4 output
function beta_i_node_4 = fcn(k_2_ij_vec, err_wi_vec)
%%%% 计算障碍函数偏导数
iiuav = 4;
beta_i_node_4 = zeros(3,1);
for jj = 1:3
%     beta_i_node_4(jj) = ( 1 / k_2_ij_vec(jj,iiuav) ) * ( 1 / ( cos( (pi/2) * ( err_wi_vec(jj,iiuav) / k_2_ij_vec(jj,iiuav) ) ) ^ 2 ) );
    beta_i_node_4(jj) = ( 1 / k_2_ij_vec(jj,iiuav) ) * ( pi / 2 ) * ( 1 / ( cos( (pi/2) * ( err_wi_vec(jj,iiuav) / k_2_ij_vec(jj,iiuav) ) ) ^ 2 ) );
end

== matlab function sim_tase_2025_att_ctrl/cal beta_i agent 5 ==
  data: k_2_ij_vec input; err_wi_vec input; beta_i_node_5 output
function beta_i_node_5 = fcn(k_2_ij_vec, err_wi_vec)
%%%% 计算障碍函数偏导数
iiuav = 5;
beta_i_node_5 = zeros(3,1);
for jj = 1:3
%     beta_i_node_5(jj) = ( 1 / k_2_ij_vec(jj,iiuav) ) * ( 1 / ( cos( (pi/2) * ( err_wi_vec(jj,iiuav) / k_2_ij_vec(jj,iiuav) ) ) ^ 2 ) );
    beta_i_node_5(jj) = ( 1 / k_2_ij_vec(jj,iiuav) ) * ( pi / 2 ) * ( 1 / ( cos( (pi/2) * ( err_wi_vec(jj,iiuav) / k_2_ij_vec(jj,iiuav) ) ) ^ 2 ) );
end

== matlab function sim_tase_2025_att_ctrl/combine beta_i ==
  data: beta_i_node_1 input; beta_i_vec output; beta_i_node_2 input; beta_i_node_3 input; beta_i_node_4 input; beta_i_node_5 input
function beta_i_vec = fcn(beta_i_node_1, beta_i_node_2, beta_i_node_3, beta_i_node_4, beta_i_node_5)
%%%% 合并障碍函数偏导数
beta_i_vec = [beta_i_node_1(:), beta_i_node_2(:), beta_i_node_3(:), beta_i_node_4(:), beta_i_node_5(:)];

== matlab function sim_tase_2025_att_ctrl/cal taui agent 2 ==
  data: c2 input; beta_i_vec input; eta_2_ij_vec input; tau_2 output; dw_hat_vec input
function tau_2 = fcn(c2, beta_i_vec, eta_2_ij_vec, dw_hat_vec)
%%%% 计算用于姿态控制的驱动力矩控制输入
iiuav = 2;
tau_2 = -c2 * beta_i_vec(:,iiuav) .* eta_2_ij_vec(:,iiuav) - dw_hat_vec(:,iiuav);
end

== matlab function sim_tase_2025_att_ctrl/depart Qc2 ==
  data: y output; x input
function y = fcn(x)
y = x(:,2);

end

== matlab function sim_tase_2025_att_ctrl/cal taui agent 3 ==
  data: c2 input; beta_i_vec input; eta_2_ij_vec input; tau_3 output; dw_hat_vec input
function tau_3 = fcn(c2, beta_i_vec, eta_2_ij_vec, dw_hat_vec)
%%%% 计算用于姿态控制的驱动力矩控制输入
iiuav = 3;
tau_3 = -c2 * beta_i_vec(:,iiuav) .* eta_2_ij_vec(:,iiuav) - dw_hat_vec(:,iiuav);
end

== matlab function sim_tase_2025_att_ctrl/cal taui agent 4 ==
  data: c2 input; beta_i_vec input; eta_2_ij_vec input; tau_4 output; dw_hat_vec input
function tau_4 = fcn(c2, beta_i_vec, eta_2_ij_vec, dw_hat_vec)
%%%% 计算用于姿态控制的驱动力矩控制输入
iiuav = 4;
tau_4 = -c2 * beta_i_vec(:,iiuav) .* eta_2_ij_vec(:,iiuav) - dw_hat_vec(:,iiuav);
end

== matlab function sim_tase_2025_att_ctrl/cal taui agent 5 ==
  data: c2 input; beta_i_vec input; eta_2_ij_vec input; tau_5 output; dw_hat_vec input
function tau_5 = fcn(c2, beta_i_vec, eta_2_ij_vec, dw_hat_vec)
%%%% 计算用于姿态控制的驱动力矩控制输入
iiuav = 5;
tau_5 = -c2 * beta_i_vec(:,iiuav) .* eta_2_ij_vec(:,iiuav) - dw_hat_vec(:,iiuav);
end

== matlab function sim_tase_2025_att_ctrl/depart k_2_ij 5 ==
  data: y output; x input
function y = fcn(x)
y = x(:,5);

end

== matlab function sim_tase_2025_att_ctrl/depart k_2_ij 1 ==
  data: y output; x input
function y = fcn(x)
y = x(:,1);

end

== matlab function sim_tase_2025_att_ctrl/depart k_2_ij 2 ==
  data: y output; x input
function y = fcn(x)
y = x(:,2);

end

== matlab function sim_tase_2025_att_ctrl/depart k_2_ij 3 ==
  data: y output; x input
function y = fcn(x)
y = x(:,3);

end

== matlab function sim_tase_2025_att_ctrl/depart k_2_ij 4 ==
  data: y output; x input
function y = fcn(x)
y = x(:,4);

end

== matlab function sim_tase_2025_att_ctrl/depart Qc3 ==
  data: y output; x input
function y = fcn(x)
y = x(:,3);

end

== matlab function sim_tase_2025_att_ctrl/depart err_wi 5 ==
  data: y output; x input
function y = fcn(x)
y = x(:,5);

end

== matlab function sim_tase_2025_att_ctrl/depart err_wi 1 ==
  data: y output; x input
function y = fcn(x)
y = x(:,1);

end

== matlab function sim_tase_2025_att_ctrl/depart err_wi 2 ==
  data: y output; x input
function y = fcn(x)
y = x(:,2);

end

== matlab function sim_tase_2025_att_ctrl/depart err_wi 3 ==
  data: y output; x input
function y = fcn(x)
y = x(:,3);

end

== matlab function sim_tase_2025_att_ctrl/depart err_wi 4 ==
  data: y output; x input
function y = fcn(x)
y = x(:,4);

end

== matlab function sim_tase_2025_att_ctrl/cal combine sigma_bar_w_tilt ==
  data: sigma_bar_w_vec input; sigma_bar_w_hat_vec input; sigma_bar_w_tilt_vec output
function sigma_bar_w_tilt_vec = fcn(sigma_bar_w_vec, sigma_bar_w_hat_vec)
%%%% 计算虚拟速度观测误差sigma_bar_w_tilt
sigma_bar_w_tilt_vec = zeros(3,5);
for iiuav = 1:5
    sigma_bar_w_tilt_vec(:,iiuav) = sigma_bar_w_vec(:,iiuav) - sigma_bar_w_hat_vec(:,iiuav);
end

== matlab function sim_tase_2025_att_ctrl/cal differentiator d_sigma_bar_w_hat agent 3/cal sig3 ==
  data: x input; z output; y input
function z = fcn(x, y)
z = x(:) .* sign(y(:));

== matlab function sim_tase_2025_att_ctrl/cal differentiator d_sigma_bar_w_hat agent 3/cal sig4 ==
  data: x input; z output; y input
function z = fcn(x, y)
z = x(:) .* sign(y(:));

== matlab function sim_tase_2025_att_ctrl/cal wei agent 1 ==
  data: wi_vec input; wei_1 output; Rei_vec input; wci_vec input
function wei_1 = fcn(wi_vec, Rei_vec, wci_vec)
%%%% 更新姿态角速率误差
iiuav = 1;
wei_1 = wi_vec(:,iiuav) - (Rei_vec(:,:,iiuav)') * wci_vec(:,iiuav);

end

== matlab function sim_tase_2025_att_ctrl/Qei dynam agent 1 ==
  data: Qei_vec input; dQei_1 output; wei_vec input
function dQei_1 = fcn(Qei_vec, wei_vec)
%%%% 更新四元数误差微分方程
iiuav = 1;

wei = wei_vec(:,iiuav);
thetaei = Qei_vec(1,iiuav);
qei = Qei_vec(2:4,iiuav);

GammaQei = zeros(4,3);
GammaQei(1,:) = -(qei');
GammaQei(2:4,:) = thetaei*eye(3,3) + cal_askew_mat(qei);
dQei_1 = (1/2)*GammaQei*wei;

end

== matlab function sim_tase_2025_att_ctrl/depart Qc4 ==
  data: y output; x input
function y = fcn(x)
y = x(:,4);

end

== matlab function sim_tase_2025_att_ctrl/cal Rei agent 1 ==
  data: Rei_1 output; Qei_vec input
function Rei_1 = fcn(Qei_vec)
%%%% 使用罗德里格公式由四元数Qei求解Rei
iiuav = 1;
thetaei_tmp = Qei_vec(1,iiuav);
qei_tmp = Qei_vec(2:4,iiuav);
Rei_1 = ((thetaei_tmp^2) - (qei_tmp')*qei_tmp) * eye(3,3) ...
                + 2 * qei_tmp * (qei_tmp') ...
                - 2 * thetaei_tmp * cal_askew_mat(qei_tmp);

end

== matlab function sim_tase_2025_att_ctrl/Qei dynam agent 2 ==
  data: Qei_vec input; dQei_2 output; wei_vec input
function dQei_2 = fcn(Qei_vec, wei_vec)
%%%% 更新四元数误差微分方程
iiuav = 2;

wei = wei_vec(:,iiuav);
thetaei = Qei_vec(1,iiuav);
qei = Qei_vec(2:4,iiuav);

GammaQei = zeros(4,3);
GammaQei(1,:) = -(qei');
GammaQei(2:4,:) = thetaei*eye(3,3) + cal_askew_mat(qei);
dQei_2 = (1/2)*GammaQei*wei;

end

== matlab function sim_tase_2025_att_ctrl/cal differentiator d_sigma_bar_w_hat agent 3/cal sig5 ==
  data: x input; z output; y input
function z = fcn(x, y)
z = x(:) .* sign(y(:));

== matlab function sim_tase_2025_att_ctrl/cal Rei agent 2 ==
  data: Rei_2 output; Qei_vec input
function Rei_2 = fcn(Qei_vec)
%%%% 使用罗德里格公式由四元数Qei求解Rei
iiuav = 2;
thetaei_tmp = Qei_vec(1,iiuav);
qei_tmp = Qei_vec(2:4,iiuav);
Rei_2 = ((thetaei_tmp^2) - (qei_tmp')*qei_tmp) * eye(3,3) ...
                + 2 * qei_tmp * (qei_tmp') ...
                - 2 * thetaei_tmp * cal_askew_mat(qei_tmp);

end

== matlab function sim_tase_2025_att_ctrl/cal wei agent 2 ==
  data: wi_vec input; wei_2 output; Rei_vec input; wci_vec input
function wei_2 = fcn(wi_vec, Rei_vec, wci_vec)
%%%% 更新姿态角速率误差
iiuav = 2;
wei_2 = wi_vec(:,iiuav) - (Rei_vec(:,:,iiuav)') * wci_vec(:,iiuav);

end

== matlab function sim_tase_2025_att_ctrl/Qei dynam agent 3 ==
  data: Qei_vec input; dQei_3 output; wei_vec input
function dQei_3 = fcn(Qei_vec, wei_vec)
%%%% 更新四元数误差微分方程
iiuav = 3;

wei = wei_vec(:,iiuav);
thetaei = Qei_vec(1,iiuav);
qei = Qei_vec(2:4,iiuav);

GammaQei = zeros(4,3);
GammaQei(1,:) = -(qei');
GammaQei(2:4,:) = thetaei*eye(3,3) + cal_askew_mat(qei);
dQei_3 = (1/2)*GammaQei*wei;

end

== matlab function sim_tase_2025_att_ctrl/cal Rei agent 3 ==
  data: Rei_3 output; Qei_vec input
function Rei_3 = fcn(Qei_vec)
%%%% 使用罗德里格公式由四元数Qei求解Rei
iiuav = 3;
thetaei_tmp = Qei_vec(1,iiuav);
qei_tmp = Qei_vec(2:4,iiuav);
Rei_3 = ((thetaei_tmp^2) - (qei_tmp')*qei_tmp) * eye(3,3) ...
                + 2 * qei_tmp * (qei_tmp') ...
                - 2 * thetaei_tmp * cal_askew_mat(qei_tmp);

end

== matlab function sim_tase_2025_att_ctrl/cal wei agent 3 ==
  data: wi_vec input; wei_3 output; Rei_vec input; wci_vec input
function wei_3 = fcn(wi_vec, Rei_vec, wci_vec)
%%%% 更新姿态角速率误差
iiuav = 3;
wei_3 = wi_vec(:,iiuav) - (Rei_vec(:,:,iiuav)') * wci_vec(:,iiuav);

end

== matlab function sim_tase_2025_att_ctrl/cal phi_ij agent 5 ==
  data: tsim input; phi_ij_5 output; T_ij input
function phi_ij_5 = fcn(tsim, T_ij)
%%%% 计算性能调节函数
iiuav = 5;
phi_ij_5 = zeros(3,1);
for jj = 1:3
%     kk_phi = 1.0;
%     phi_ij_5(jj) = 1 - sin( (pi/2) * ( ( kk_phi * tsim ) / ( T_ij(jj, iiuav) ) ) );
%     if phi_ij_5(jj) < 0
%         phi_ij_5(jj) = 0;
%     end

    kk_phi = 1.0;
    if tsim <= T_ij(jj, iiuav)
        phi_ij_5(jj) = 1 - sin( (pi/2) * ( ( kk_phi * tsim ) / ( T_ij(jj, iiuav) ) ) );
    else
        phi_ij_5(jj) = 0;
    end

end

== matlab function sim_tase_2025_att_ctrl/Qei dynam agent 4 ==
  data: Qei_vec input; dQei_4 output; wei_vec input
function dQei_4 = fcn(Qei_vec, wei_vec)
%%%% 更新四元数误差微分方程
iiuav = 4;

wei = wei_vec(:,iiuav);
thetaei = Qei_vec(1,iiuav);
qei = Qei_vec(2:4,iiuav);

GammaQei = zeros(4,3);
GammaQei(1,:) = -(qei');
GammaQei(2:4,:) = thetaei*eye(3,3) + cal_askew_mat(qei);
dQei_4 = (1/2)*GammaQei*wei;

end

== matlab function sim_tase_2025_att_ctrl/cal Rei agent 4 ==
  data: Rei_4 output; Qei_vec input
function Rei_4 = fcn(Qei_vec)
%%%% 使用罗德里格公式由四元数Qei求解Rei
iiuav = 4;
thetaei_tmp = Qei_vec(1,iiuav);
qei_tmp = Qei_vec(2:4,iiuav);
Rei_4 = ((thetaei_tmp^2) - (qei_tmp')*qei_tmp) * eye(3,3) ...
                + 2 * qei_tmp * (qei_tmp') ...
                - 2 * thetaei_tmp * cal_askew_mat(qei_tmp);

end

== matlab function sim_tase_2025_att_ctrl/cal wei agent 4 ==
  data: wi_vec input; wei_4 output; Rei_vec input; wci_vec input
function wei_4 = fcn(wi_vec, Rei_vec, wci_vec)
%%%% 更新姿态角速率误差
iiuav = 4;
wei_4 = wi_vec(:,iiuav) - (Rei_vec(:,:,iiuav)') * wci_vec(:,iiuav);

end

== matlab function sim_tase_2025_att_ctrl/Qei dynam agent 5 ==
  data: Qei_vec input; dQei_5 output; wei_vec input
function dQei_5 = fcn(Qei_vec, wei_vec)
%%%% 更新四元数误差微分方程
iiuav = 5;

wei = wei_vec(:,iiuav);
thetaei = Qei_vec(1,iiuav);
qei = Qei_vec(2:4,iiuav);

GammaQei = zeros(4,3);
GammaQei(1,:) = -(qei');
GammaQei(2:4,:) = thetaei*eye(3,3) + cal_askew_mat(qei);
dQei_5 = (1/2)*GammaQei*wei;

end

== matlab function sim_tase_2025_att_ctrl/cal Rei agent 5 ==
  data: Rei_5 output; Qei_vec input
function Rei_5 = fcn(Qei_vec)
%%%% 使用罗德里格公式由四元数Qei求解Rei
iiuav = 5;
thetaei_tmp = Qei_vec(1,iiuav);
qei_tmp = Qei_vec(2:4,iiuav);
Rei_5 = ((thetaei_tmp^2) - (qei_tmp')*qei_tmp) * eye(3,3) ...
                + 2 * qei_tmp * (qei_tmp') ...
                - 2 * thetaei_tmp * cal_askew_mat(qei_tmp);

end

== matlab function sim_tase_2025_att_ctrl/cal wei agent 5 ==
  data: wi_vec input; wei_5 output; Rei_vec input; wci_vec input
function wei_5 = fcn(wi_vec, Rei_vec, wci_vec)
%%%% 更新姿态角速率误差
iiuav = 5;
wei_5 = wi_vec(:,iiuav) - (Rei_vec(:,:,iiuav)') * wci_vec(:,iiuav);

end
